simulink model "Kalition"  (R2016a)
settings: Solver=ode2  StartTime=0.0  StopTime=10.0  FixedStep=0.01  RelTol=1e-3
InitFcn:
  | Parameters
settings Model: Creator=pela  LastModifiedBy=ergae
settings DataIOCC: LimitDataPoints=on  SaveFormat=Array
settings HardwareCC: ProdBitPerPointer=32  ProdLargestAtomicInteger=Long  ProdLargestAtomicFloat=Double  ProdIntDivRoundTo=Undefined  ProdWordSize=32  ProdHWDeviceType=ARM Compatible->ARM Cortex
settings ModelReferenceCC: PropagateSignalLabelsOutOfModel=off
settings RTWCC: GenCodeOnly=on  GenerateReport=on  Toolchain=Microsoft Visual C++ 2013 v12.0 | nmake (64-bit Windows)  BuildConfiguration=Faster Runs  LaunchReport=on  TargetLang=C++
settings GRTTargetCC: MatFileLogging=off  MultiInstanceERTCode=on  CodeInterfacePackaging=C++ class  SupportNonFinite=off
settings ConfigComp: CovModelRefEnable=Off

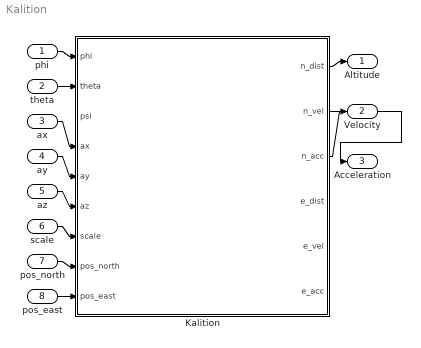
== system Kalition ==
  phi : Inport
  theta : Inport  Port=2
  ax : Inport  Port=3
  ay : Inport  Port=4
  az : Inport  Port=5
  scale : Inport  Port=6
  pos_north : Inport  Port=7
  pos_east : Inport  Port=8
  Kalition : Subsystem
  Altitude : Outport
  Velocity : Outport  Port=2
  Acceleration : Outport  Port=3
  wires:
  phi/1 -> Kalition/1(phi)
  theta/1 -> Kalition/2(theta)
  ax/1 -> Kalition/4(ax)
  ay/1 -> Kalition/5(ay)
  Kalition/1(n_dist) -> Altitude/1
  Kalition/3(n_acc) -> Velocity/1
  Kalition/2(n_vel) -> Acceleration/1
  az/1 -> Kalition/6(az)
  scale/1 -> Kalition/7(scale)
  pos_north/1 -> Kalition/8(pos_north)
  pos_east/1 -> Kalition/9(pos_east)

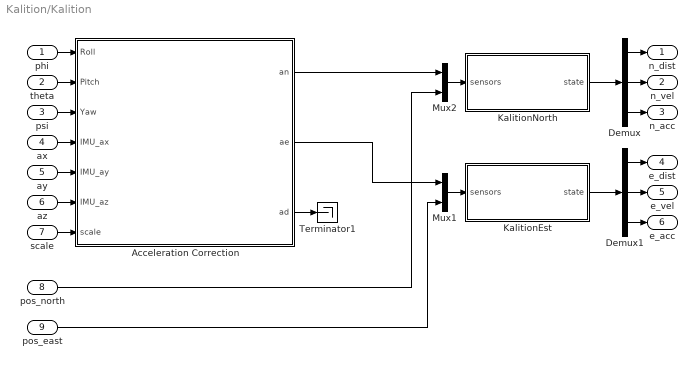
== system Kalition/Kalition ==
  phi : Inport
  theta : Inport  Port=2
  psi : Inport  Port=3
  ax : Inport  Port=4
  ay : Inport  Port=5
  az : Inport  Port=6
  scale : Inport  Port=7
  pos_north : Inport  Port=8
  pos_east : Inport  Port=9
  Acceleration Correction : MATLAB Function  TreatAsAtomicUnit=on
  Demux : Demux  Outputs=3
  Demux1 : Demux  Outputs=3
  KalitionEst : Subsystem
  KalitionNorth : Subsystem
  Mux1 : Mux  Inputs=2
  Mux2 : Mux  Inputs=2
  Terminator1 : Terminator
  n_dist : Outport
  n_vel : Outport  Port=2
  n_acc : Outport  Port=3
  e_dist : Outport  Port=4
  e_vel : Outport  Port=5
  e_acc : Outport  Port=6
  wires:
  ax/1 -> Acceleration Correction/4(IMU_ax)
  phi/1 -> Acceleration Correction/1(Roll)
  theta/1 -> Acceleration Correction/2(Pitch)
  Mux1/1 -> KalitionEst/1(sensors)
  ay/1 -> Acceleration Correction/5(IMU_ay)
  Acceleration Correction/1(an) -> Mux2/1
  KalitionEst/1(state) -> Demux1/1
  Demux/1 -> n_dist/1
  Demux/2 -> n_vel/1
  Demux/3 -> n_acc/1
  az/1 -> Acceleration Correction/6(IMU_az)
  scale/1 -> Acceleration Correction/7(scale)
  pos_north/1 -> Mux2/2
  Acceleration Correction/2(ae) -> Mux1/1
  Mux2/1 -> KalitionNorth/1(sensors)
  Acceleration Correction/3(ad) -> Terminator1/1
  pos_east/1 -> Mux1/2
  psi/1 -> Acceleration Correction/3(Yaw)
  KalitionNorth/1(state) -> Demux/1
  Demux1/1 -> e_dist/1
  Demux1/2 -> e_vel/1
  Demux1/3 -> e_acc/1

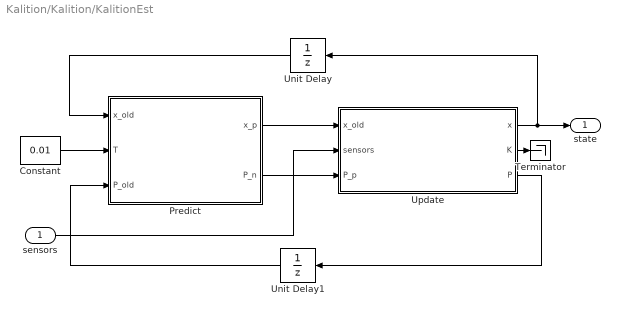
== system Kalition/Kalition/KalitionEst ==
  sensors : Inport
  Constant : Constant  Value=0.01  VectorParams1D=off  SampleTime=-1
  "Predict " : MATLAB Function  TreatAsAtomicUnit=on
  Terminator : Terminator
  Unit Delay : UnitDelay  InitialCondition=zeros(3,1)  SampleTime=-1
  Unit Delay1 : UnitDelay  InitialCondition=eye(3)*0.001  SampleTime=-1
  Update : MATLAB Function  TreatAsAtomicUnit=on
  state : Outport
  wires:
  Update/2(K) -> Terminator/1
  Unit Delay1/1 -> "Predict "/3(P_old)
  Update/1(x) -> state/1, Unit Delay/1
  "Predict "/1(x_p) -> Update/1(x_old)
  sensors/1 -> Update/2(sensors)
  "Predict "/2(P_n) -> Update/3(P_p)
  Constant/1 -> "Predict "/2(T)
  Update/3(P) -> Unit Delay1/1
  Unit Delay/1 -> "Predict "/1(x_old)

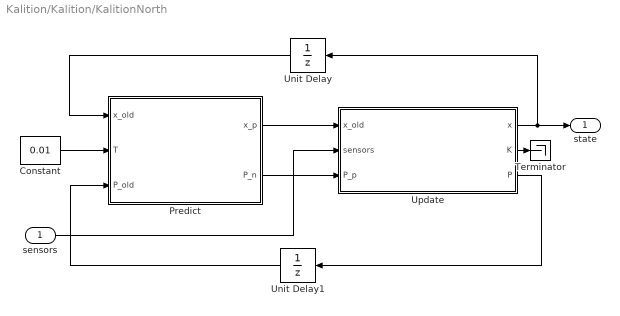
== system Kalition/Kalition/KalitionNorth ==
  sensors : Inport
  Constant : Constant  Value=0.01  VectorParams1D=off  SampleTime=-1
  "Predict " : MATLAB Function  TreatAsAtomicUnit=on
  Terminator : Terminator
  Unit Delay : UnitDelay  InitialCondition=zeros(3,1)  SampleTime=-1
  Unit Delay1 : UnitDelay  InitialCondition=eye(3)*0.001  SampleTime=-1
  Update : MATLAB Function  TreatAsAtomicUnit=on
  state : Outport
  wires:
  Unit Delay/1 -> "Predict "/1(x_old)
  Update/3(P) -> Unit Delay1/1
  Constant/1 -> "Predict "/2(T)
  "Predict "/2(P_n) -> Update/3(P_p)
  sensors/1 -> Update/2(sensors)
  "Predict "/1(x_p) -> Update/1(x_old)
  Update/1(x) -> Unit Delay/1, state/1
  Unit Delay1/1 -> "Predict "/3(P_old)
  Update/2(K) -> Terminator/1

== matlab function Kalition/KalitionNorth/Predict  ==
  data x_old settings: description=State estimate at the previous step.
  data x_p settings: description=A-priori state estimate.
  data T settings: description=Control signal at the previous step.
  data P_n settings: description=A-priori covariance estimate.
  data P_old settings: description=Covariance estimate at the previous step.
  data: x_old input; x_p output; T input; P_n output; P_old input
%%AKF state update        %
% Author: Matteo Ferronato%
% Last review: 2016/05/23 %
%%%%%%%%%%%%%%%%%%%%%%%%%%%
function [x_p,P_n] = state_predict(x_old,T,P_old)
%% State-noise matrix
Qn = [0.005   0     0   ;
        0   0.005   0   ;
        0     0   0.005];

%% Dynamics matrix
A = [ 1, T, T^2/2;
      0,   1,   T;
      0,   0,   1];

x_p = A*x_old;

%% Covariance propagation
P_n = A*P_old*A' + Qn;

== matlab function Kalition/Acceleration Correction ==
  data: an output; ae output; ad output; Roll input; Pitch input; Yaw input; IMU_ax input; IMU_ay input; IMU_az input; scale input
function [an,ae,ad] = Accelerometer_correction(Roll,Pitch,Yaw,IMU_ax,IMU_ay,IMU_az,scale)
%#codegen
acc_norm_x = IMU_ax/scale;
a_corr_x = sqrt(sin(Roll)^2 + sin(Pitch)^2);
acc_norm_y = IMU_ay/scale;
a_corr_y = sqrt(sin(Roll)^2 + sin(Pitch)^2);
acc_norm_z = IMU_az/scale;
a_corr_z = sqrt(1 - (sin(Roll)^2 + sin(Pitch)^2));

ax = (acc_norm_x + a_corr_x)*9.81;
ay=(acc_norm_y + a_corr_y)*9.81;
az = (acc_norm_z - a_corr_z)*9.81;

Rot=[cos(Yaw) sin(Yaw);
-sin(Yaw) cos(Yaw)];
Aned = Rot*[ax ay]';
an = Aned(1);
ae = Aned(2);
ad = az;

== matlab function Kalition/KalitionNorth/Update ==
  data x_old settings: description=A-priori state estimate.
  data sensors settings: description=Measurements from the sensors.
  data x settings: description=Corrected state estimate.
  data P_p settings: description=A-priori covariance estimate.
  data P settings: description=Corrected covariance estimate.
  data: x_old input; sensors input; x output; K output; P_p input; P output
%%A-KF state correction   %
% Author: Matteo Ferronato%
% Last review: 2016/05/23 %
%%%%%%%%%%%%%%%%%%%%%%%%%%%
function [x,K,P] = state_update(x_old,sensors,P_p)
% Useful Parameters
Rn = [1    0 ;
      0   0.7];
%%
H = [1 0 0 ;
     0 0 1 ];

%%
h = H*x_old;

%%
Pl = P_p;
x_p = x_old;

for j = 1:2
    % Innovation covariance
    S = H(j,:)*Pl*H(j,:)' + Rn(j,j);
    
    % Kalman gain
    K = Pl*H(j,:)'/S;
    
    % Updated state estimate
    x_p = x_p + K*(sensors(j,1)-h(j,1));
    
    % Updated estimated covariance
    Pl = (eye(3) - K*H(j,:))*Pl*(eye(3) - K*H(j,:))' + K*Rn(j,j)*K';
end

P = Pl;
x = x_p;

== matlab function Kalition/KalitionEst/Update ==
  data x_old settings: description=A-priori state estimate.
  data sensors settings: description=Measurements from the sensors.
  data x settings: description=Corrected state estimate.
  data P_p settings: description=A-priori covariance estimate.
  data P settings: description=Corrected covariance estimate.
  data: x_old input; sensors input; x output; K output; P_p input; P output
%%A-KF state correction   %
% Author: Matteo Ferronato%
% Last review: 2016/05/23 %
%%%%%%%%%%%%%%%%%%%%%%%%%%%
function [x,K,P] = state_update(x_old,sensors,P_p)
% Useful Parameters
Rn = [1    0 ;
      0   0.7];
%%
H = [1 0 0 ;
     0 0 1 ];

%%
h = H*x_old;

%%
Pl = P_p;
x_p = x_old;

for j = 1:2
    % Innovation covariance
    S = H(j,:)*Pl*H(j,:)' + Rn(j,j);
    
    % Kalman gain
    K = Pl*H(j,:)'/S;
    
    % Updated state estimate
    x_p = x_p + K*(sensors(j,1)-h(j,1));
    
    % Updated estimated covariance
    Pl = (eye(3) - K*H(j,:))*Pl*(eye(3) - K*H(j,:))' + K*Rn(j,j)*K';
end

P = Pl;
x = x_p;

== matlab function Kalition/KalitionEst/Predict  ==
  data x_old settings: description=State estimate at the previous step.
  data x_p settings: description=A-priori state estimate.
  data T settings: description=Control signal at the previous step.
  data P_n settings: description=A-priori covariance estimate.
  data P_old settings: description=Covariance estimate at the previous step.
  data: x_old input; x_p output; T input; P_n output; P_old input
%%AKF state update        %
% Author: Matteo Ferronato%
% Last review: 2016/05/23 %
%%%%%%%%%%%%%%%%%%%%%%%%%%%
function [x_p,P_n] = state_predict(x_old,T,P_old)
%% State-noise matrix
Qn = [0.005   0     0   ;
        0   0.005   0   ;
        0     0   0.005];

%% Dynamics matrix
A = [ 1, T, T^2/2;
      0,   1,   T;
      0,   0,   1];

x_p = A*x_old;

%% Covariance propagation
P_n = A*P_old*A' + Qn;
